simulink model "Navion_6DoF_10_auto_ascend_2023"  (R2024a)
settings: Solver=ode45  StartTime=0.0  StopTime=500  FixedStep=.01  MaxStep=.004  RelTol=1e-5  EnableMultiTasking=on
values from neighbouring files (symbols this model uses):
  ac = [0 0 0]    [Navion_Geom_temp.m]
  b = 33.4    [Navion_Geom_temp.m]
  cbar = 5.7    [Navion_Geom_temp.m]
  cda2 = 0.33    [Navion_Geom_temp.m]
  cdo = 0.05    [Navion_Geom_temp.m]
  cg = [0 0 0]    [Navion_Geom_temp.m]
  cla = 4.44    [Navion_Geom_temp.m]
  cladot = 0    [Navion_Geom_temp.m]
  clb = -0.074    [Navion_Geom_temp.m]
  clda = -0.134    [Navion_Geom_temp.m]
  clde = 0.355    [Navion_Geom_temp.m]
  cldr = 0.107    [Navion_Geom_temp.m]
  clo = 0.41    [Navion_Geom_temp.m]
  clp = -0.410    (= -0.41)    [Navion_Geom_temp.m]
  clq = 3.8    [Navion_Geom_temp.m]
  clr = 0.107    [Navion_Geom_temp.m]
  cma = -0.683    [Navion_Geom_temp.m]
  cmadot = -4.36    [Navion_Geom_temp.m]
  cmde = -0.923    [Navion_Geom_temp.m]
  cmq = -9.96    [Navion_Geom_temp.m]
  cnb = 0.071    [Navion_Geom_temp.m]
  cnda = -0.0035    [Navion_Geom_temp.m]
  cndr = -0.072    [Navion_Geom_temp.m]
  cnp = -0.0575    [Navion_Geom_temp.m]
  cnr = -0.125    [Navion_Geom_temp.m]
  cyb = -0.564    [Navion_Geom_temp.m]
  cydr = 0.157    [Navion_Geom_temp.m]
  eng = [0 0 0]    [Navion_Geom_temp.m]
  initalt = 5000    [Navion_Geom_temp.m]
  initbank = 0    [Navion_Geom_temp.m]
  initeast = 0    [Navion_Geom_temp.m]
  inithead = 0    [Navion_Geom_temp.m]
  initnorth = 0    [Navion_Geom_temp.m]
  initp = 0    [Navion_Geom_temp.m]
  initpitch = initw/initu    (= 0)    [Navion_Geom_temp.m]
  initq = 0    [Navion_Geom_temp.m]
  initr = 0    [Navion_Geom_temp.m]
  initu = 223    [Navion_Geom_temp.m]
  initv = 0    [Navion_Geom_temp.m]
  initw = 0    [Navion_Geom_temp.m]
  jx = 1048    [Navion_Geom_temp.m]
  jxz = 0    [Navion_Geom_temp.m]
  jy = 3000    [Navion_Geom_temp.m]
  jz = 3500    [Navion_Geom_temp.m]
  sw = 184    [Navion_Geom_temp.m]
  weight = 2750    [Navion_Geom_temp.m]
undefined symbols (not defined in the file or in its folder): Earth, WGS84
libraries: simulink_extras x9, slpidlib x6, aerolibfltsims x2, simulink x2, aerolibtransform2 x1, aerolibanimutils x1
(part 2 of 2)

== system Navion_6DoF_10_auto_ascend_2023/longitudinal autopilot/Descend ==
  note: this is desired rate of climb
  R/C : Inport
  Action Port : ActionPort  ActionPortLabel=elseif(u1 <100)
  Debugging : Constant  Value=2
  PID Controller : slpidlib/PID Controller  Controller=PID  Form=Parallel  TimeDomain=Continuous-time  UseExternalTs=off  SampleTime=-1  IntegratorMethod=Forward Euler  FilterMethod=Forward Euler  ControllerParametersSource=internal  P=1  I=1  UseKiTs=off  D=0  N=100  UseFilter=on  TunerSelectOption=Transfer Function Based (PID Tuner App)  InitialConditionSource=internal  InitialConditionForIntegrator=0  InitialConditionForFilter=0  DifferentiatorICPrevScaledInput=0  ExternalReset=none  TrackingMode=off  Kt=1  LimitOutput=off  SatLimitsSource=internal  UpperSaturationLimit=inf  LowerSaturationLimit=-inf  LinearizeAsGain=on  AntiWindupMode=none  Kb=1  LimitIntegrator=off  UpperIntegratorSaturationLimit=inf  LowerIntegratorSaturationLimit=-inf  POutMin=[]  POutMax=[]  IOutMin=[]  IOutMax=[]  DOutMin=[]  DOutMax=[]  NOutMin=[]  NOutMax=[]  SumOutMin=[]  SumOutMax=[]  SaturationOutMin=[]  SaturationOutMax=[]  PParamMin=[]  PParamMax=[]  IParamMin=[]  IParamMax=[]  DParamMin=[]  DParamMax=[]  NParamMin=[]  NParamMax=[]  KbParamMin=[]  KbParamMax=[]  KtParamMin=[]  KtParamMax=[]  KbOutMin=[]  KbOutMax=[]  KtOutMin=[]  KtOutMax=[]  IntegratorOutMin=[]  IntegratorOutMax=[]  FilterOutMin=[]  FilterOutMax=[]  SumI1OutMin=[]  SumI1OutMax=[]  SumI2OutMin=[]  SumI2OutMax=[]  SumI3OutMin=[]  SumI3OutMax=[]  SumI4OutMin=[]  SumI4OutMax=[]  SumDOutMin=[]  SumDOutMax=[]  DifferentiatorOutMin=[]  DifferentiatorOutMax=[]  FilterDiffOutCoefMin=[]  FilterDiffOutCoefMax=[]  ReciprocalOutMin=[]  ReciprocalOutMax=[]  SumDenOutMin=[]  SumDenOutMax=[]  SumNumOutMin=[]  SumNumOutMax=[]  DivideOutMin=[]  DivideOutMax=[]  UdiffTsProdOutMin=[]  UdiffTsProdOutMax=[]  NTsProdOutMin=[]  NTsProdOutMax=[]  UintegralTsProdOutMin=[]  UintegralTsProdOutMax=[]  UngainTsProdOutMin=[]  UngainTsProdOutMax=[]  ClampingZeroOutDataTypeStr=Inherit: Inherit via back propagation  ClampingZeroOutMin=[]  ClampingZeroOutMax=[]  FilterDenConstantOutDataTypeStr=Inherit: Inherit via back propagation  FilterDenConstantOutMin=[]  FilterDenConstantOutMax=[]  PCopyOutDataTypeStr=Inherit: Inherit via back propagation  PCopyOutMin=[]  PCopyOutMax=[]  NCopyOutDataTypeStr=Inherit: Inherit via back propagation  NCopyOutMin=[]  NCopyOutMax=[]  IntegratorContinuousStateAttributes=''  IntegratorStateMustResolveToSignalObject=off  IntegratorRTWStateStorageClass=Auto  FilterContinuousStateAttributes=''  FilterStateMustResolveToSignalObject=off  FilterRTWStateStorageClass=Auto  ParallelPVariant=InternalParameters  IdealPVariant=Disabled  IVariant=InternalParameters  DVariant=InternalParameters  IntegratorVariant=Continuous  SatVariant=Disabled  AWVariant=Passthrough  PCopyVariant=Disabled  TRVariant=Disabled  FdbkBlocksVariant=Forward  IdealPFdbkVariant=Disabled  SatFdbkVariant=Disabled  DerivativeFilterVariant=ContFilter  NVariant=InternalParameters  NCopyVariant=Disabled  FilterICVariant=InternalICsFilter  IntegratorICVariant=InternalICs  ExternalResetVariant=Disabled  TRSumVariant=Passthrough  SumFdbkVariant=Disabled  SumVariant=Sum_PID  TsampFilterVariant=InternalTs  TsampNgainVariant=Passthrough  TsampIntegralVariant=Disabled_SignalSpec  ExternalSaturationOutDataTypeStr=Inherit: Same as second input
  R/C_CMD : Constant  Value=-1
  Sum : Sum  Inputs=|+-
  del_e_auto : Outport
  Debug : Outport  Port=2
  wires:
  Debugging/1 -> Debug/1
  R/C_CMD/1 -> Sum/2
  PID Controller/1 -> del_e_auto/1
  Sum/1 -> PID Controller/1
  R/C/1 -> Sum/1

== system Navion_6DoF_10_auto_ascend_2023/longitudinal autopilot/Level ==
  h_err : Inport
  Action Port : ActionPort  ActionPortLabel=else
  Constant : Constant  Value=3
  PID Controller : slpidlib/PID Controller  Controller=PID  Form=Parallel  TimeDomain=Continuous-time  UseExternalTs=off  SampleTime=-1  IntegratorMethod=Forward Euler  FilterMethod=Forward Euler  ControllerParametersSource=internal  P=8.53679546434618e-05  I=3.54615014998628e-06  UseKiTs=off  D=0.000510671209456043  N=32.652227886903  UseFilter=on  TunerSelectOption=Transfer Function Based (PID Tuner App)  InitialConditionSource=internal  InitialConditionForIntegrator=0  InitialConditionForFilter=0  DifferentiatorICPrevScaledInput=0  ExternalReset=none  TrackingMode=off  Kt=1  LimitOutput=on  SatLimitsSource=internal  UpperSaturationLimit=.4363  LowerSaturationLimit=-.4363  LinearizeAsGain=off  AntiWindupMode=none  Kb=1  LimitIntegrator=off  UpperIntegratorSaturationLimit=inf  LowerIntegratorSaturationLimit=-inf  POutMin=[]  POutMax=[]  IOutMin=[]  IOutMax=[]  DOutMin=[]  DOutMax=[]  NOutMin=[]  NOutMax=[]  SumOutMin=[]  SumOutMax=[]  SaturationOutMin=[]  SaturationOutMax=[]  PParamMin=[]  PParamMax=[]  IParamMin=[]  IParamMax=[]  DParamMin=[]  DParamMax=[]  NParamMin=[]  NParamMax=[]  KbParamMin=[]  KbParamMax=[]  KtParamMin=[]  KtParamMax=[]  KbOutMin=[]  KbOutMax=[]  KtOutMin=[]  KtOutMax=[]  IntegratorOutMin=[]  IntegratorOutMax=[]  FilterOutMin=[]  FilterOutMax=[]  SumI1OutMin=[]  SumI1OutMax=[]  SumI2OutMin=[]  SumI2OutMax=[]  SumI3OutMin=[]  SumI3OutMax=[]  SumI4OutMin=[]  SumI4OutMax=[]  SumDOutMin=[]  SumDOutMax=[]  DifferentiatorOutMin=[]  DifferentiatorOutMax=[]  FilterDiffOutCoefMin=[]  FilterDiffOutCoefMax=[]  ReciprocalOutMin=[]  ReciprocalOutMax=[]  SumDenOutMin=[]  SumDenOutMax=[]  SumNumOutMin=[]  SumNumOutMax=[]  DivideOutMin=[]  DivideOutMax=[]  UdiffTsProdOutMin=[]  UdiffTsProdOutMax=[]  NTsProdOutMin=[]  NTsProdOutMax=[]  UintegralTsProdOutMin=[]  UintegralTsProdOutMax=[]  UngainTsProdOutMin=[]  UngainTsProdOutMax=[]  ClampingZeroOutDataTypeStr=Inherit: Inherit via back propagation  ClampingZeroOutMin=[]  ClampingZeroOutMax=[]  FilterDenConstantOutDataTypeStr=Inherit: Inherit via back propagation  FilterDenConstantOutMin=[]  FilterDenConstantOutMax=[]  PCopyOutDataTypeStr=Inherit: Inherit via back propagation  PCopyOutMin=[]  PCopyOutMax=[]  NCopyOutDataTypeStr=Inherit: Inherit via back propagation  NCopyOutMin=[]  NCopyOutMax=[]  IntegratorContinuousStateAttributes=''  IntegratorStateMustResolveToSignalObject=off  IntegratorRTWStateStorageClass=Auto  FilterContinuousStateAttributes=''  FilterStateMustResolveToSignalObject=off  FilterRTWStateStorageClass=Auto  ParallelPVariant=InternalParameters  IdealPVariant=Disabled  IVariant=InternalParameters  DVariant=InternalParameters  IntegratorVariant=Continuous  SatVariant=Enabled  AWVariant=Passthrough  PCopyVariant=Disabled  TRVariant=Disabled  FdbkBlocksVariant=Forward  IdealPFdbkVariant=Disabled  SatFdbkVariant=Disabled  DerivativeFilterVariant=ContFilter  NVariant=InternalParameters  NCopyVariant=Disabled  FilterICVariant=InternalICsFilter  IntegratorICVariant=InternalICs  ExternalResetVariant=Disabled  TRSumVariant=Passthrough  SumFdbkVariant=Disabled  SumVariant=Sum_PID  TsampFilterVariant=InternalTs  TsampNgainVariant=Passthrough  TsampIntegralVariant=Disabled_SignalSpec  ExternalSaturationOutDataTypeStr=Inherit: Same as second input
  del_e_auto : Outport
  Debug : Outport  Port=2
  wires:
  h_err/1 -> PID Controller/1
  PID Controller/1 -> del_e_auto/1  "Hal"
  Constant/1 -> Debug/1

== system Navion_6DoF_10_auto_ascend_2023/Aircraft_Dynamics/Aerodynamics/Aero Forces and Moments ==
  dyn(q) : Inport
  CD : Inport  Port=2
  CY : Inport  Port=3
  CL : Inport  Port=4
  Wind Para : Inport  Port=5
  Croll : Inport  Port=6
  CM : Inport  Port=7
  CN : Inport  Port=8
  Aerodynamic Forces : Subsystem
  Aerodynamic Moments : Subsystem
  Faero : Outport
  Maero : Outport  Port=2
  wires:
  dyn(q)/1 -> Aerodynamic Moments/1(dyn(q)), Aerodynamic Forces/5(dyn(q))
  CD/1 -> Aerodynamic Forces/1(CD)
  CY/1 -> Aerodynamic Forces/2(CY)
  CL/1 -> Aerodynamic Forces/3(CL)
  Wind Para/1 -> Aerodynamic Forces/4(Wind Para)
  Croll/1 -> Aerodynamic Moments/2(Croll)
  CM/1 -> Aerodynamic Moments/3(CM)
  CN/1 -> Aerodynamic Moments/4(CN)
  Aerodynamic Forces/1(FaeroBody) -> Faero/1
  Aerodynamic Moments/1(Maero) -> Maero/1

== system Navion_6DoF_10_auto_ascend_2023/Aircraft_Dynamics/Aerodynamics/CD ==
  Wind Parameters : Inport
  Controls : Inport  Port=2
  Mach No. : Inport  Port=3
  "   1" : Terminator
  "   6" : Terminator
  Get Alpha : Subsystem
  Math Function : Math  Operator=square  SignedPower=on
  Sum : Sum  SaturateOnIntegerOverflow=on
  cda2 : Gain  Gain=cda2  SaturateOnIntegerOverflow=on  OutDataTypeStr=Inherit: Same as input  ParamDataTypeStr=Inherit: Same as input
  cdo : Constant  Value=cdo
  CD : Outport
  wires:
  Wind Parameters/1 -> Get Alpha/1(windPar)
  Sum/1 -> CD/1
  Controls/1 -> "   6"/1
  Get Alpha/1(Alpha) -> Math Function/1
  Math Function/1 -> cda2/1
  cda2/1 -> Sum/2
  Mach No./1 -> "   1"/1
  cdo/1 -> Sum/1

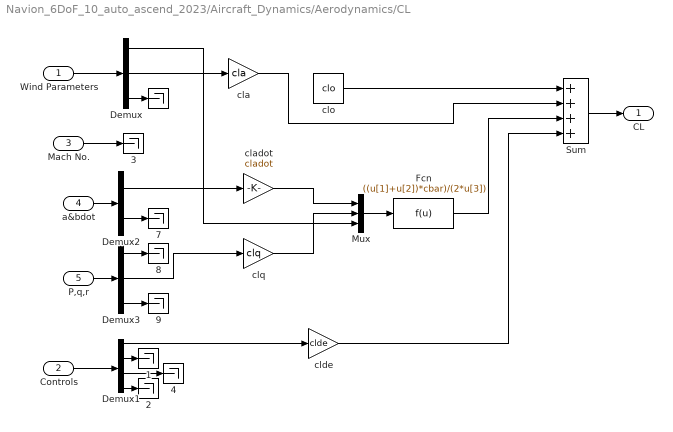
== system Navion_6DoF_10_auto_ascend_2023/Aircraft_Dynamics/Aerodynamics/CL ==
  Wind Parameters : Inport
  Controls : Inport  Port=2
  Mach No. : Inport  Port=3
  a&bdot : Inport  Port=4
  P,q,r : Inport  Port=5
     {,1..4,7..9} (8 alike) : Terminator
  Demux : Demux  Outputs=3
      settings: DisplayOption=none
  Demux1 : Demux
      settings: DisplayOption=none
  Demux2 : Demux  Outputs=2
      settings: DisplayOption=none
  Demux3 : Demux  Outputs=3
      settings: DisplayOption=none
  Fcn : Fcn  Expr=((u[1]+u[2])*cbar)/(2*u[3])
  Mux : Mux  Inputs=3
  Sum : Sum  Inputs=++++  SaturateOnIntegerOverflow=on
  cla : Gain  Gain=cla  SaturateOnIntegerOverflow=on  OutDataTypeStr=Inherit: Same as input  ParamDataTypeStr=Inherit: Same as input
  cladot : Gain  Gain=cladot  SaturateOnIntegerOverflow=on  OutDataTypeStr=Inherit: Same as input  ParamDataTypeStr=Inherit: Same as input
  clde : Gain  Gain=clde  SaturateOnIntegerOverflow=on  OutDataTypeStr=Inherit: Same as input  ParamDataTypeStr=Inherit: Same as input
  clo : Constant  Value=clo
  clq : Gain  Gain=clq  SaturateOnIntegerOverflow=on  OutDataTypeStr=Inherit: Same as input  ParamDataTypeStr=Inherit: Same as input
  CL : Outport
  wires:
  Mux/1 -> Fcn/1
  Demux/1 -> Mux/3
  clo/1 -> Sum/1
  Demux2/2 -> "   7"/1
  Demux3/1 -> "   8"/1
  Demux3/3 -> "   9"/1
  Wind Parameters/1 -> Demux/1
  Sum/1 -> CL/1
  Controls/1 -> Demux1/1
  a&bdot/1 -> Demux2/1
  P,q,r/1 -> Demux3/1
  Demux/3 -> "   "/1
  Demux1/4 -> "   2"/1
  cla/1 -> Sum/2
  Demux2/1 -> cladot/1
  cladot/1 -> Mux/1
  Demux/2 -> cla/1
  clq/1 -> Mux/2
  Mach No./1 -> "   3"/1
  Demux3/2 -> clq/1
  Demux1/1 -> clde/1
  Demux1/2 -> "   1"/1
  Demux1/3 -> "   4"/1
  Fcn/1 -> Sum/3
  clde/1 -> Sum/4

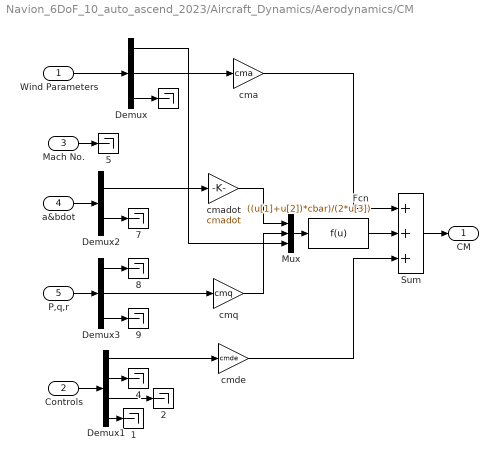
== system Navion_6DoF_10_auto_ascend_2023/Aircraft_Dynamics/Aerodynamics/CM ==
  Wind Parameters : Inport
  Controls : Inport  Port=2
  Mach No. : Inport  Port=3
  a&bdot : Inport  Port=4
  P,q,r : Inport  Port=5
     {,1..2,4..5,7..9} (8 alike) : Terminator
  Demux : Demux  Outputs=3
      settings: DisplayOption=none
  Demux1 : Demux
      settings: DisplayOption=none
  Demux2 : Demux  Outputs=2
      settings: DisplayOption=none
  Demux3 : Demux  Outputs=3
      settings: DisplayOption=none
  Fcn : Fcn  Expr=((u[1]+u[2])*cbar)/(2*u[3])
  Mux : Mux  Inputs=3
  Sum : Sum  Inputs=+++  SaturateOnIntegerOverflow=on
  cma : Gain  Gain=cma  SaturateOnIntegerOverflow=on  OutDataTypeStr=Inherit: Same as input  ParamDataTypeStr=Inherit: Same as input
  cmadot : Gain  Gain=cmadot  SaturateOnIntegerOverflow=on  OutDataTypeStr=Inherit: Same as input  ParamDataTypeStr=Inherit: Same as input
  cmde : Gain  Gain=cmde  SaturateOnIntegerOverflow=on  OutDataTypeStr=Inherit: Same as input  ParamDataTypeStr=Inherit: Same as input
  cmq : Gain  Gain=cmq  SaturateOnIntegerOverflow=on  OutDataTypeStr=Inherit: Same as input  ParamDataTypeStr=Inherit: Same as input
  CM : Outport
  wires:
  Demux2/2 -> "   7"/1
  Demux3/1 -> "   8"/1
  Demux3/3 -> "   9"/1
  Wind Parameters/1 -> Demux/1
  Sum/1 -> CM/1
  Controls/1 -> Demux1/1
  a&bdot/1 -> Demux2/1
  P,q,r/1 -> Demux3/1
  Demux/3 -> "   "/1
  Demux1/4 -> "   1"/1
  Demux1/3 -> "   2"/1
  Demux/2 -> cma/1
  cmadot/1 -> Mux/1
  cmq/1 -> Mux/2
  Mux/1 -> Fcn/1
  Demux1/2 -> "   4"/1
  Mach No./1 -> "   5"/1
  Demux/1 -> Mux/3
  cma/1 -> Sum/1
  Demux1/1 -> cmde/1
  Demux2/1 -> cmadot/1
  Demux3/2 -> cmq/1
  Fcn/1 -> Sum/2
  cmde/1 -> Sum/3

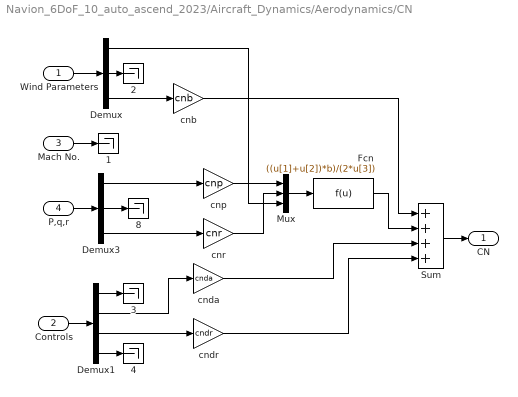
== system Navion_6DoF_10_auto_ascend_2023/Aircraft_Dynamics/Aerodynamics/CN ==
  Wind Parameters : Inport
  Controls : Inport  Port=2
  Mach No. : Inport  Port=3
  P,q,r : Inport  Port=4
     {1..4,8} (5 alike) : Terminator
  Demux : Demux  Outputs=3
      settings: DisplayOption=none
  Demux1 : Demux
      settings: DisplayOption=none
  Demux3 : Demux  Outputs=3
      settings: DisplayOption=none
  Fcn : Fcn  Expr=((u[1]+u[2])*b)/(2*u[3])
  Mux : Mux  Inputs=3
  Sum : Sum  Inputs=++++  SaturateOnIntegerOverflow=on
  cnb : Gain  Gain=cnb  SaturateOnIntegerOverflow=on  OutDataTypeStr=Inherit: Same as input  ParamDataTypeStr=Inherit: Same as input
  cnda : Gain  Gain=cnda  SaturateOnIntegerOverflow=on  OutDataTypeStr=Inherit: Same as input  ParamDataTypeStr=Inherit: Same as input
  cndr : Gain  Gain=cndr  SaturateOnIntegerOverflow=on  OutDataTypeStr=Inherit: Same as input  ParamDataTypeStr=Inherit: Same as input
  cnp : Gain  Gain=cnp  SaturateOnIntegerOverflow=on  OutDataTypeStr=Inherit: Same as input  ParamDataTypeStr=Inherit: Same as input
  cnr : Gain  Gain=cnr  SaturateOnIntegerOverflow=on  OutDataTypeStr=Inherit: Same as input  ParamDataTypeStr=Inherit: Same as input
  CN : Outport
  wires:
  Mux/1 -> Fcn/1
  Demux/2 -> "   2"/1
  Wind Parameters/1 -> Demux/1
  Sum/1 -> CN/1
  Controls/1 -> Demux1/1
  P,q,r/1 -> Demux3/1
  Demux3/2 -> "   8"/1
  cnb/1 -> Sum/1
  Mach No./1 -> "   1"/1
  Demux/3 -> cnb/1
  Demux/1 -> Mux/3
  Demux3/1 -> cnp/1
  cnp/1 -> Mux/1
  Demux3/3 -> cnr/1
  cnr/1 -> Mux/2
  Demux1/2 -> cnda/1
  Demux1/3 -> cndr/1
  Fcn/1 -> Sum/2
  cnda/1 -> Sum/3
  cndr/1 -> Sum/4
  Demux1/1 -> "   3"/1
  Demux1/4 -> "   4"/1

== system Navion_6DoF_10_auto_ascend_2023/Aircraft_Dynamics/Aerodynamics/CY ==
  Wind Parameters : Inport
  Controls : Inport  Port=2
  Mach No. : Inport  Port=3
  P,q,r : Inport  Port=4
     {2,7..12} (7 alike) : Terminator
  Demux : Demux  Outputs=3
      settings: DisplayOption=none
  Demux1 : Demux
      settings: DisplayOption=none
  Sum : Sum  SaturateOnIntegerOverflow=on
  cyb : Gain  Gain=cyb  SaturateOnIntegerOverflow=on  OutDataTypeStr=Inherit: Same as input  ParamDataTypeStr=Inherit: Same as input
  cydr : Gain  Gain=cydr  SaturateOnIntegerOverflow=on  OutDataTypeStr=Inherit: Same as input  ParamDataTypeStr=Inherit: Same as input
  CY : Outport
  wires:
  Demux/2 -> "   9"/1
  Wind Parameters/1 -> Demux/1
  Sum/1 -> CY/1
  Controls/1 -> Demux1/1
  P,q,r/1 -> "   8"/1
  Demux/3 -> cyb/1
  Mach No./1 -> "   2"/1
  Demux1/3 -> cydr/1
  Demux1/1 -> "   10"/1
  Demux1/2 -> "   7"/1
  Demux1/4 -> "   11"/1
  cyb/1 -> Sum/1
  cydr/1 -> Sum/2
  Demux/1 -> "   12"/1

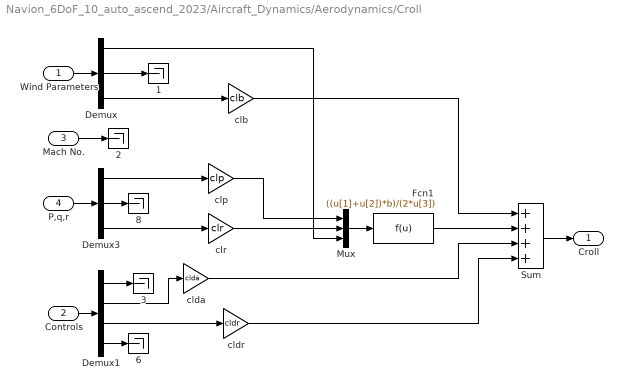
== system Navion_6DoF_10_auto_ascend_2023/Aircraft_Dynamics/Aerodynamics/Croll ==
  Wind Parameters : Inport
  Controls : Inport  Port=2
  Mach No. : Inport  Port=3
  P,q,r : Inport  Port=4
     {1..3,6,8} (5 alike) : Terminator
  Demux : Demux  Outputs=3
      settings: DisplayOption=none
  Demux1 : Demux
      settings: DisplayOption=none
  Demux3 : Demux  Outputs=3
      settings: DisplayOption=none
  Fcn1 : Fcn  Expr=((u[1]+u[2])*b)/(2*u[3])
  Mux : Mux  Inputs=3
  Sum : Sum  Inputs=++++  SaturateOnIntegerOverflow=on
  clb : Gain  Gain=clb  SaturateOnIntegerOverflow=on  OutDataTypeStr=Inherit: Same as input  ParamDataTypeStr=Inherit: Same as input
  clda : Gain  Gain=clda  SaturateOnIntegerOverflow=on  OutDataTypeStr=Inherit: Same as input  ParamDataTypeStr=Inherit: Same as input
  cldr : Gain  Gain=cldr  SaturateOnIntegerOverflow=on  OutDataTypeStr=Inherit: Same as input  ParamDataTypeStr=Inherit: Same as input
  clp : Gain  Gain=clp  SaturateOnIntegerOverflow=on  OutDataTypeStr=Inherit: Same as input  ParamDataTypeStr=Inherit: Same as input
  clr : Gain  Gain=clr  SaturateOnIntegerOverflow=on  OutDataTypeStr=Inherit: Same as input  ParamDataTypeStr=Inherit: Same as input
  Croll : Outport
  wires:
  Mux/1 -> Fcn1/1
  Demux/2 -> "   1"/1
  Wind Parameters/1 -> Demux/1
  Sum/1 -> Croll/1
  Controls/1 -> Demux1/1
  P,q,r/1 -> Demux3/1
  Demux3/2 -> "   8"/1
  Demux1/1 -> "   3"/1
  clp/1 -> Mux/1
  clb/1 -> Sum/1
  Demux/1 -> Mux/3
  Demux/3 -> clb/1
  Mach No./1 -> "   2"/1
  Demux3/1 -> clp/1
  Fcn1/1 -> Sum/2
  Demux3/3 -> clr/1
  clr/1 -> Mux/2
  Demux1/4 -> "   6"/1
  Demux1/2 -> clda/1
  Demux1/3 -> cldr/1
  clda/1 -> Sum/3
  cldr/1 -> Sum/4

== system Navion_6DoF_10_auto_ascend_2023/Aircraft_Dynamics/Equations of motion numerical integration /Flat Earth Navigation ==
  note: 1  roll
      | 2  pitch
      | 3  yaw
      | 4 u
      | 5 v
      | 6 w
  Euler Angles : Inport
  Velocity : Inport  Port=2
  Alt : Integrator  InitialCondition=initalt
  Alttitude Dot : Fcn  Expr=u[4] * sin(u[2]) - u[5] * sin(u[1]) * cos(u[2]) - u[6] * cos(u[1]) * cos(u[2])
  Demux : Demux  Outputs=3
      settings: DisplayOption=none
  Demux1 : Demux  Outputs=3
      settings: DisplayOption=none
  East : Integrator  InitialCondition=initeast
  East Dot : Fcn  Expr=u[4] * cos(u[2])* sin(u[3]) + u[5] * (cos(u[1])*cos(u[3]) + sin(u[1])*sin(u[2])*sin(u[3])) + u[6] * (-sin(u[1])*cos(u[3])+cos(u[1])*sin(u[2])*sin(u[3]))
  Mux : Mux  Inputs=6
  Mux1 : Mux  Inputs=3
  North : Integrator  InitialCondition=initnorth
  North Dot : Fcn  Expr=u[4] * cos(u[2]) * cos(u[3]) + u[5]*(-cos(u[1])*sin(u[3])+sin(u[1])*sin(u[2])*sin(u[3]))+u[6]*(sin(u[1])*sin(u[3])+cos(u[1])*sin(u[2])*cos(u[3]))
  Position : Outport
  R/C : Outport  Port=2
  wires:
  Euler Angles/1 -> Demux/1
  Velocity/1 -> Demux1/1
  Demux/1 -> Mux/1
  Demux/2 -> Mux/2
  Demux/3 -> Mux/3
  Demux1/1 -> Mux/4
  Demux1/2 -> Mux/5
  Demux1/3 -> Mux/6
  Mux/1 -> East Dot/1, Alttitude Dot/1, North Dot/1
  East Dot/1 -> East/1
  North Dot/1 -> North/1
  Alttitude Dot/1 -> R/C/1, Alt/1
  East/1 -> Mux1/2
  North/1 -> Mux1/1
  Alt/1 -> Mux1/3
  Mux1/1 -> Position/1

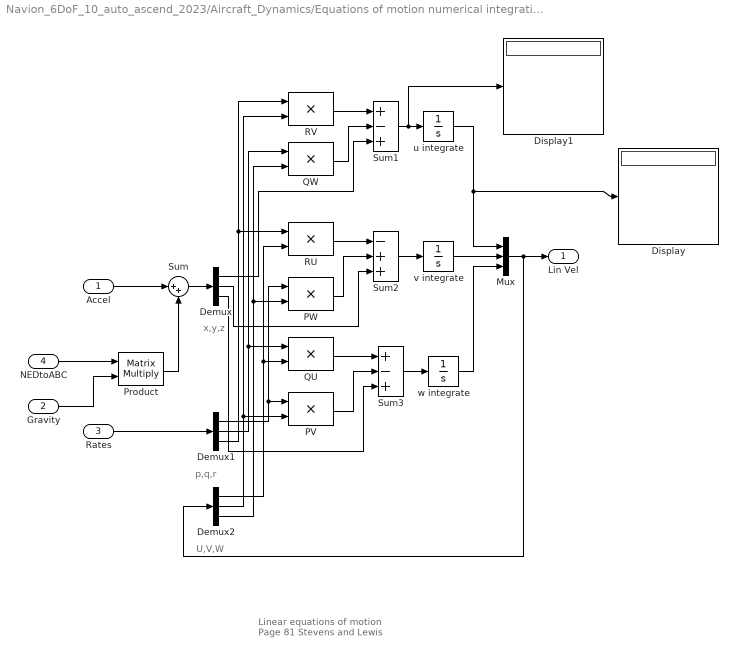
== system Navion_6DoF_10_auto_ascend_2023/Aircraft_Dynamics/Equations of motion numerical integration /Force Equations ==
  note: U,V,W
  note: p,q,r
  note: x,y,z
  note: Linear equations of motion
      | Page 81 Stevens and Lewis
  Accel : Inport
  Gravity : Inport  Port=2
  Rates : Inport  Port=3
  NEDtoABC : Inport  Port=4
  Demux : Demux  Outputs=3
      settings: DisplayOption=none
  Demux1 : Demux  Outputs=3
      settings: DisplayOption=none
  Demux2 : Demux  Outputs=3
      settings: DisplayOption=none
  Display : Display
  Display1 : Display
  Mux : Mux  Inputs=3
  PV : Product  SaturateOnIntegerOverflow=on  OutDataTypeStr=Inherit: Same as first input
  PW : Product  SaturateOnIntegerOverflow=on  OutDataTypeStr=Inherit: Same as first input
  Product : Product  Multiplication=Matrix(*)  SaturateOnIntegerOverflow=on  OutDataTypeStr=Inherit: Same as first input
  QU : Product  SaturateOnIntegerOverflow=on  OutDataTypeStr=Inherit: Same as first input
  QW : Product  SaturateOnIntegerOverflow=on  OutDataTypeStr=Inherit: Same as first input
  RU : Product  SaturateOnIntegerOverflow=on  OutDataTypeStr=Inherit: Same as first input
  RV : Product  SaturateOnIntegerOverflow=on  OutDataTypeStr=Inherit: Same as first input
  Sum : Sum  Inputs=|++  SaturateOnIntegerOverflow=on
  Sum1 : Sum  Inputs=+-+  SaturateOnIntegerOverflow=on
  Sum2 : Sum  Inputs=-++  SaturateOnIntegerOverflow=on
  Sum3 : Sum  Inputs=+-+  SaturateOnIntegerOverflow=on
  u integrate : Integrator  InitialCondition=initu
  v integrate : Integrator  InitialCondition=initv
  w integrate : Integrator  InitialCondition=initw
  Lin Vel : Outport
  wires:
  Sum/1 -> Demux/1
  Accel/1 -> Sum/1
  Rates/1 -> Demux1/1
  Mux/1 -> Demux2/1, Lin Vel/1
  Demux1/3 -> RV/1, RU/1
  Demux2/2 -> RV/2, PV/2
  RV/1 -> Sum1/1
  Demux1/2 -> QW/1, QU/1
  Demux2/3 -> QW/2, PW/2
  QW/1 -> Sum1/2
  Demux/1 -> Sum1/3
  Demux2/1 -> RU/2, QU/2
  RU/1 -> Sum2/1
  Demux1/1 -> PV/1, PW/1
  PW/1 -> Sum2/2
  Demux/2 -> Sum2/3
  QU/1 -> Sum3/1
  PV/1 -> Sum3/2
  Demux/3 -> Sum3/3
  Gravity/1 -> Product/2
  NEDtoABC/1 -> Product/1
  Product/1 -> Sum/2
  Sum1/1 -> u integrate/1, Display1/1
  Sum2/1 -> v integrate/1
  Sum3/1 -> w integrate/1
  u integrate/1 -> Mux/1, Display/1
  v integrate/1 -> Mux/2
  w integrate/1 -> Mux/3

== system Navion_6DoF_10_auto_ascend_2023/Aircraft_Dynamics/Equations of motion numerical integration /Gravity Model ==
  Constant : Constant  Value=0
  Constant1 : Constant  Value=32.2
  Mux : Mux  Inputs=3
  Gravity : Outport
  wires:
  Constant/1 -> Mux/1, Mux/2
  Constant1/1 -> Mux/3
  Mux/1 -> Gravity/1

== system Navion_6DoF_10_auto_ascend_2023/Aircraft_Dynamics/Equations of motion numerical integration /Inert-body ==
  Euler : Inport
  11 : Fcn  Expr=cos(u[2])*cos(u[3])
  12 : Fcn  Expr=-cos(u[1])*sin(u[3])+sin(u[1])*sin(u[2])*cos(u[3])
  13 : Fcn  Expr=sin(u[1])*sin(u[3])+cos(u[1])*sin(u[2])*cos(u[3])
  21 : Fcn  Expr=cos(u[2])*sin(u[3])
  22 : Fcn  Expr=cos(u[1])*cos(u[3]) + sin(u[1])*sin(u[2])*sin(u[3])
  23 : Fcn  Expr=-sin(u[1])*cos(u[3])+cos(u[1])*sin(u[2])*sin(u[3])
  31 : Fcn  Expr=-sin(u[2])
  32 : Fcn  Expr=sin(u[1]) * cos(u[2])
  33 : Fcn  Expr=cos(u[1])*cos(u[2])
  Matrix Concatenation : Concatenate  NumInputs=3  Mode=Multidimensional array
  Matrix Concatenation1 : Concatenate  NumInputs=3  Mode=Multidimensional array
  Matrix Concatenation2 : Concatenate  NumInputs=3  Mode=Multidimensional array
  Matrix Concatenation3 : Concatenate  NumInputs=3  Mode=Multidimensional array  ConcatenateDimension=2
  NEDtoBC : Outport
  wires:
  Euler/1 -> 11/1, 12/1, 13/1, 21/1, 22/1, 23/1, 31/1, 33/1, 32/1
  12/1 -> Matrix Concatenation/2
  11/1 -> Matrix Concatenation/1
  13/1 -> Matrix Concatenation/3
  22/1 -> Matrix Concatenation1/2
  21/1 -> Matrix Concatenation1/1
  23/1 -> Matrix Concatenation1/3
  32/1 -> Matrix Concatenation2/2
  31/1 -> Matrix Concatenation2/1
  33/1 -> Matrix Concatenation2/3
  Matrix Concatenation1/1 -> Matrix Concatenation3/2
  Matrix Concatenation/1 -> Matrix Concatenation3/1
  Matrix Concatenation2/1 -> Matrix Concatenation3/3
  Matrix Concatenation3/1 -> NEDtoBC/1

== system Navion_6DoF_10_auto_ascend_2023/Aircraft_Dynamics/Equations of motion numerical integration /Kinematic Equiations ==
  note: 1  p
      | 2  q
      | 3  r
      | 4  bank
      | 5 pitch
      | 6 Yaw
  Rates : Inport
  2pi Bound : Subsystem  mask(2pi bound){}
      mask help: Bounds the input angle to [0, 2pi]. When 0 bound is exceeded the output wraps back to 2pi; when the 2pi bound is exceeded the output wraps back to 0.
      mask Help:
      | Bounds the input angle to [0, 2pi]. When 0 bound is exceeded the output wraps back to 2pi; when the 2pi bound is exceeded the output wraps back to 0.
      | <P><B>Input:</B> any angle in radians, from -Inf to Inf;</P>
      | <P><B>Output:</B> an angle in radians between zero and 2pi.</P>
  Demux : Demux  Outputs=3
      settings: DisplayOption=none
  Demux1 : Demux  Outputs=3
      settings: DisplayOption=none
  Demux2 : Demux  Outputs=3
      settings: DisplayOption=none
  Mux : Mux  Inputs=6
  Mux1 : Mux  Inputs=3
  Mux2 : Mux  Inputs=3
  Yaw rate : Fcn  Expr=(u[2] * sin(u[4]) + u[3] * cos(u[4]))/cos(u[5])
  bank : Integrator  InitialCondition=initbank
  heading : Integrator  InitialCondition=inithead
  pi Bound : Subsystem  mask(pi bound){}
      mask help: Bounds the input angle to [-pi, pi]. When -pi bound is exceeded the output wraps back to pi; when the pi bound is exceeded the output wraps back to -pi.
      mask Help:
      | Bounds the input angle to [-pi, pi]. When -pi bound is exceeded the output wraps back to pi; when the pi bound is exceeded the output wraps back to -pi.
      | <P><B>Input:</B> any angle in radians, from -Inf to Inf;</P>
      | <P><B>Output:</B> an angle in radians between -pi and pi.</P>
  pi Bound1 : Subsystem  mask(pi bound){}
      mask help: Bounds the input angle to [-pi, pi]. When -pi bound is exceeded the output wraps back to pi; when the pi bound is exceeded the output wraps back to -pi.
      mask Help:
      | Bounds the input angle to [-pi, pi]. When -pi bound is exceeded the output wraps back to pi; when the pi bound is exceeded the output wraps back to -pi.
      | <P><B>Input:</B> any angle in radians, from -Inf to Inf;</P>
      | <P><B>Output:</B> an angle in radians between -pi and pi.</P>
  pitch : Integrator  InitialCondition=initpitch
  pitch rate : Fcn  Expr=u[2] *cos(u[4]) - u[3] * sin(u[4])
  roll rate : Fcn  Expr=u[1] + tan(u[5])*(u[2]*sin(u[4])+u[3]*cos(u[4]))
  Euler angles : Outport
  wires:
  Rates/1 -> Demux/1
  Demux/2 -> Mux/2
  Demux/3 -> Mux/3
  Demux1/1 -> Mux/4
  Demux1/2 -> Mux/5
  Demux1/3 -> Mux/6
  Demux/1 -> Mux/1
  Mux/1 -> roll rate/1, Yaw rate/1, pitch rate/1
  Demux2/3 -> 2pi Bound/1(In)
  Demux2/2 -> pi Bound/1(In)
  Demux2/1 -> pi Bound1/1(In)
  Mux2/1 -> Euler angles/1
  pi Bound/1(Out) -> Mux2/2
  pi Bound1/1(Out) -> Mux2/1
  2pi Bound/1(Out) -> Mux2/3
  pitch rate/1 -> pitch/1
  roll rate/1 -> bank/1
  Yaw rate/1 -> heading/1
  bank/1 -> Mux1/1
  pitch/1 -> Mux1/2
  heading/1 -> Mux1/3
  Mux1/1 -> Demux2/1, Demux1/1

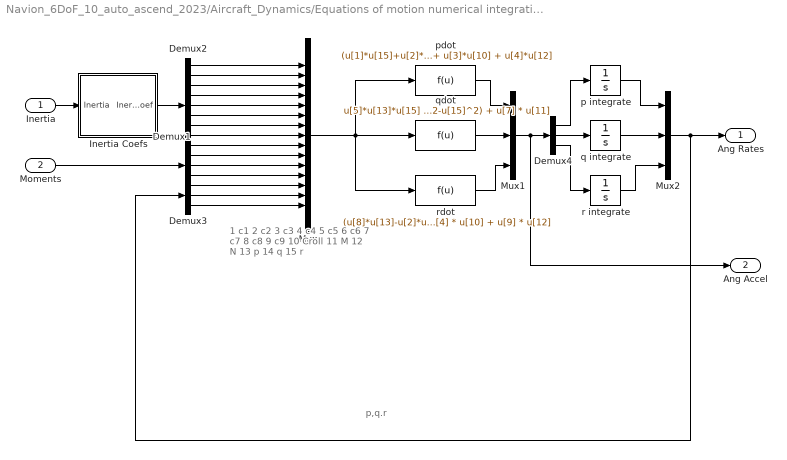
== system Navion_6DoF_10_auto_ascend_2023/Aircraft_Dynamics/Equations of motion numerical integration /Moment Equations ==
  note: 1   c1
      | 2   c2
      | 3   c3
      | 4  c4
      | 5  c5
      | 6  c6
      | 7  c7
      | 8  c8
      | 9  c9
      | 10 Croll
      | 11  M
      | 12  N
      | 13  p
      | 14  q
      | 15  r
  note: p,q.r
  Inertia : Inport
  Moments : Inport  Port=2
  Demux1 : Demux  Outputs=3
      settings: DisplayOption=none
  Demux2 : Demux  Outputs=9
      settings: DisplayOption=none
  Demux3 : Demux  Outputs=3
      settings: DisplayOption=none
  Demux4 : Demux  Outputs=3
      settings: DisplayOption=none
  Inertia Coefs : Subsystem
  Mux : Mux  Inputs=15
  Mux1 : Mux  Inputs=3
  Mux2 : Mux  Inputs=3
  p integrate : Integrator  InitialCondition=initp
  pdot : Fcn  Expr=(u[1]*u[15]+u[2]*u[13])*u[14] + u[3]*u[10] + u[4]*u[12]
  q integrate : Integrator  InitialCondition=initq
  qdot : Fcn  Expr=u[5]*u[13]*u[15] - u[6]*(u[13]^2-u[15]^2) + u[7] * u[11]
  r integrate : Integrator  InitialCondition=initr
  rdot : Fcn  Expr=(u[8]*u[13]-u[2]*u[15]) * u[14] + u[4] * u[10] + u[9] * u[12]
  Ang Rates : Outport
  Ang Accel : Outport  Port=2
  wires:
  Inertia/1 -> Inertia Coefs/1(Inertia)
  Moments/1 -> Demux1/1
  Inertia Coefs/1(Iner Coef) -> Demux2/1
  Demux2/1 -> Mux/1
  Demux2/2 -> Mux/2
  Demux2/3 -> Mux/3
  Demux2/4 -> Mux/4
  Demux2/5 -> Mux/5
  Demux2/6 -> Mux/6
  Demux2/7 -> Mux/7
  Demux2/8 -> Mux/8
  Demux2/9 -> Mux/9
  Demux1/1 -> Mux/10
  Demux1/2 -> Mux/11
  Demux1/3 -> Mux/12
  Demux3/1 -> Mux/13
  Demux3/2 -> Mux/14
  Demux3/3 -> Mux/15
  Mux/1 -> pdot/1, qdot/1, rdot/1
  qdot/1 -> Mux1/2
  pdot/1 -> Mux1/1
  rdot/1 -> Mux1/3
  Mux1/1 -> Ang Accel/1, Demux4/1
  Demux4/1 -> p integrate/1
  Demux4/2 -> q integrate/1
  Demux4/3 -> r integrate/1
  Mux2/1 -> Ang Rates/1, Demux3/1
  p integrate/1 -> Mux2/1
  q integrate/1 -> Mux2/2
  r integrate/1 -> Mux2/3

== system Navion_6DoF_10_auto_ascend_2023/Aircraft_Dynamics/Linear Acc and Moments/Cross Prod Moment due Leng ==
  Vec 1 : Inport
  Vec 2 : Inport  Port=2
  Check prob not zero : Constant  Value=0
  Demux : Demux  Outputs=3
      settings: DisplayOption=none
  J axis : Fcn  Expr=u[4]*u[3] - u[6]*u[1]
  Mux : Mux  Inputs=6
  Mux1 : Mux  Inputs=3
  i axis : Fcn  Expr=u[6]*u[2] - u[5]*u[3]
  k axis : Fcn  Expr=u[5]*u[1] - u[4]*u[2]
  X Prod : Outport
  wires:
  Vec 2/1 -> Mux/4
  Vec 1/1 -> Demux/1
  Demux/1 -> Mux/1
  Check prob not zero/1 -> Mux/5, Mux/6
  Demux/3 -> Mux/3
  Demux/2 -> Mux/2
  Mux/1 -> i axis/1, J axis/1, k axis/1
  J axis/1 -> Mux1/2
  i axis/1 -> Mux1/1
  k axis/1 -> Mux1/3
  Mux1/1 -> X Prod/1

== system Navion_6DoF_10_auto_ascend_2023/Aircraft_Dynamics/Linear Acc and Moments/Cross Prod Moment due to Aero ==
  Vec 1 : Inport
  Vec 2 : Inport  Port=2
  Demux : Demux  Outputs=3
      settings: DisplayOption=none
  Demux1 : Demux  Outputs=3
      settings: DisplayOption=none
  J axis : Fcn  Expr=u[4]*u[3] - u[6]*u[1]
  Mux : Mux  Inputs=6
  Mux1 : Mux  Inputs=3
  i axis : Fcn  Expr=u[6]*u[2] - u[5]*u[3]
  k axis : Fcn  Expr=u[5]*u[1] - u[4]*u[2]
  X Prod : Outport
  wires:
  Vec 2/1 -> Demux1/1
  Vec 1/1 -> Demux/1
  Demux/1 -> Mux/1
  Demux1/3 -> Mux/6
  Demux1/2 -> Mux/5
  Demux1/1 -> Mux/4
  Demux/3 -> Mux/3
  Demux/2 -> Mux/2
  Mux/1 -> i axis/1, J axis/1, k axis/1
  J axis/1 -> Mux1/2
  i axis/1 -> Mux1/1
  k axis/1 -> Mux1/3
  Mux1/1 -> X Prod/1

== system Navion_6DoF_10_auto_ascend_2023/Aircraft_Dynamics/Aerodynamics/Aero Forces and Moments/Aerodynamic Forces ==
  CD : Inport
  CY : Inport  Port=2
  CL : Inport  Port=3
  Wind Para : Inport  Port=4
  dyn(q) : Inport  Port=5
  Body to Wind : Subsystem
  Demux : Demux  Outputs=3
      settings: DisplayOption=none
  Gain : Gain  Gain=-1  SaturateOnIntegerOverflow=on  OutDataTypeStr=Inherit: Same as input  ParamDataTypeStr=Inherit: Same as input
  Gain1 : Gain  Gain=-1  SaturateOnIntegerOverflow=on  OutDataTypeStr=Inherit: Same as input  ParamDataTypeStr=Inherit: Same as input
  Gain2 : Gain  Gain=sw  SaturateOnIntegerOverflow=on  OutDataTypeStr=Inherit: Same as input  ParamDataTypeStr=Inherit: Same as input
  Math Function : Math  Operator=transpose  SignedPower=on
  Mux : Mux  Inputs=3
  Product : Product  SaturateOnIntegerOverflow=on  OutDataTypeStr=Inherit: Same as first input
  Product1 : Product  Multiplication=Matrix(*)  SaturateOnIntegerOverflow=on  OutDataTypeStr=Inherit: Same as first input
  Terminator : Terminator
  FaeroBody : Outport
  wires:
  Gain/1 -> Mux/1
  Gain1/1 -> Mux/3
  Mux/1 -> Product/1
  Gain2/1 -> Product/2
  CD/1 -> Gain/1
  CY/1 -> Mux/2
  CL/1 -> Gain1/1
  dyn(q)/1 -> Gain2/1
  Wind Para/1 -> Demux/1
  Demux/1 -> Terminator/1
  Body to Wind/1(Smatrix) -> Math Function/1
  Math Function/1 -> Product1/1
  Product/1 -> Product1/2
  Product1/1 -> FaeroBody/1
  Demux/2 -> Body to Wind/1(Alpha)
  Demux/3 -> Body to Wind/2(Beta)

== system Navion_6DoF_10_auto_ascend_2023/Aircraft_Dynamics/Aerodynamics/Aero Forces and Moments/Aerodynamic Moments ==
  dyn(q) : Inport
  Croll : Inport  Port=2
  CM : Inport  Port=3
  CN : Inport  Port=4
  Mux : Mux  Inputs=2
  Mux1 : Mux  Inputs=2
  Mux2 : Mux  Inputs=2
  Mux3 : Mux  Inputs=3
  Pitch : Fcn  Expr=u[1] * sw * cbar * u[2]
  Roll : Fcn  Expr=u[1] * sw * b * u[2]
  Yaw : Fcn  Expr=u[1] * sw * b * u[2]
  Maero : Outport
  wires:
  Mux/1 -> Roll/1
  Mux1/1 -> Pitch/1
  Mux2/1 -> Yaw/1
  Pitch/1 -> Mux3/2
  Roll/1 -> Mux3/1
  Yaw/1 -> Mux3/3
  dyn(q)/1 -> Mux/1, Mux1/1, Mux2/1
  Croll/1 -> Mux/2
  CM/1 -> Mux1/2
  CN/1 -> Mux2/2
  Mux3/1 -> Maero/1

== system Navion_6DoF_10_auto_ascend_2023/Aircraft_Dynamics/Aerodynamics/CD/Get Alpha ==
  windPar : Inport
  "   " : Terminator
  "   1" : Terminator
  Demux : Demux  Outputs=3
      settings: DisplayOption=none
  Alpha : Outport
  wires:
  Demux/1 -> "   1"/1
  Demux/3 -> "   "/1
  windPar/1 -> Demux/1
  Demux/2 -> Alpha/1

== system Navion_6DoF_10_auto_ascend_2023/Aircraft_Dynamics/Equations of motion numerical integration /Kinematic Equiations/2pi Bound ==
  In : Inport
  2pi : Constant  Value=2*pi
  Math Function : Math  Operator=mod  SignedPower=on
  Out : Outport
  wires:
  Math Function/1 -> Out/1
  2pi/1 -> Math Function/2
  In/1 -> Math Function/1

== system Navion_6DoF_10_auto_ascend_2023/Aircraft_Dynamics/Equations of motion numerical integration /Kinematic Equiations/pi Bound ==
  In : Inport
  2pi : Constant  Value=2*pi
  Math Function : Math  Operator=mod  SignedPower=on
  Sum1 : Sum  Inputs=|+-  InputSameDT=on  SaturateOnIntegerOverflow=on  OutDataTypeStr=Inherit: Same as first input
  Sum2 : Sum  Inputs=|++  InputSameDT=on  SaturateOnIntegerOverflow=on  OutDataTypeStr=Inherit: Same as first input
  pi : Constant  Value=pi
  Out : Outport
  wires:
  Sum1/1 -> Out/1
  pi/1 -> Sum1/2, Sum2/2
  Sum2/1 -> Math Function/1
  In/1 -> Sum2/1
  2pi/1 -> Math Function/2
  Math Function/1 -> Sum1/1

== system Navion_6DoF_10_auto_ascend_2023/Aircraft_Dynamics/Equations of motion numerical integration /Kinematic Equiations/pi Bound1 ==
  In : Inport
  2pi : Constant  Value=2*pi
  Math Function : Math  Operator=mod  SignedPower=on
  Sum1 : Sum  Inputs=|+-  InputSameDT=on  SaturateOnIntegerOverflow=on  OutDataTypeStr=Inherit: Same as first input
  Sum2 : Sum  Inputs=|++  InputSameDT=on  SaturateOnIntegerOverflow=on  OutDataTypeStr=Inherit: Same as first input
  pi : Constant  Value=pi
  Out : Outport
  wires:
  Sum1/1 -> Out/1
  pi/1 -> Sum1/2, Sum2/2
  Sum2/1 -> Math Function/1
  In/1 -> Sum2/1
  2pi/1 -> Math Function/2
  Math Function/1 -> Sum1/1

== system Navion_6DoF_10_auto_ascend_2023/Aircraft_Dynamics/Equations of motion numerical integration /Moment Equations/Inertia Coefs ==
  note: Jx,Jy,Jz,Jxz
  note: Inertia Coefficeents
      | Page 80 Stevens and Lewis
  Inertia : Inport
  Mux : Mux  Inputs=9
  c1 : Fcn  Expr=((u[2]-u[3])*u[3] - u[4]^2)/(u[1]*u[3]-u[4]^2)
  c2 : Fcn  Expr=((u[1]-u[2]+u[3])*u[4])/(u[1]*u[3]-u[4]^2)
  c3 : Fcn  Expr=u[3]/(u[1]*u[3]-u[4]^2)
  c4 : Fcn  Expr=u[4]/(u[1]*u[3]-u[4]^2)
  c5 : Fcn  Expr=(u[3]-u[1])/u[2]
  c6 : Fcn  Expr=u[4]/u[2]
  c7 : Fcn  Expr=1/u[2]
  c8 : Fcn  Expr=(u[1]*(u[1]-u[2])+u[4]^2)/(u[1]*u[3]-u[4]^2)
  c9 : Fcn  Expr=u[1]/(u[1]*u[3]-u[4]^2)
  Iner Coef : Outport
  wires:
  Inertia/1 -> c1/1, c2/1, c3/1, c4/1, c5/1, c6/1, c7/1, c9/1, c8/1
  c1/1 -> Mux/1
  c2/1 -> Mux/2
  c3/1 -> Mux/3
  c4/1 -> Mux/4
  c5/1 -> Mux/5
  c6/1 -> Mux/6
  c7/1 -> Mux/7
  c8/1 -> Mux/8
  c9/1 -> Mux/9
  Mux/1 -> Iner Coef/1

== system Navion_6DoF_10_auto_ascend_2023/Aircraft_Dynamics/Aerodynamics/Aero Forces and Moments/Aerodynamic Forces/Body to Wind ==
  note: This transforms any arbitrary vector from body axis to wind axis.
      | Page 63  Stevens and Lewis
  Alpha : Inport
  Beta : Inport  Port=2
  -ca sb : Fcn  Expr=-1 * cos(u[1]) * sin(u[2])
  -sa : Fcn  Expr=-1 * sin(u[1])
  -sa sb : Fcn  Expr="-1 * sin(u[1])  * sin(u[2])"
  Fcn8 : Fcn  Expr=cos(u[1])
  Matrix Concatenation : Concatenate  NumInputs=3  Mode=Multidimensional array
  Matrix Concatenation1 : Concatenate  NumInputs=3  Mode=Multidimensional array
  Matrix Concatenation2 : Concatenate  NumInputs=3  Mode=Multidimensional array  ConcatenateDimension=2
  Matrix Concatenation3 : Concatenate  NumInputs=3  Mode=Multidimensional array
  Mux1 : Mux  Inputs=2
  ca cb : Fcn  Expr="cos(u[1]) *  cos(u[2])"
  cb : Fcn  Expr=cos(u[2])
  sa cb : Fcn  Expr=sin(u[1]) * cos(u[2])
  sb : Fcn  Expr=sin(u[2])
  zero : Fcn  Expr=u[1] * 0
  Smatrix : Outport
  wires:
  Matrix Concatenation/1 -> Matrix Concatenation2/1
  Matrix Concatenation1/1 -> Matrix Concatenation2/2
  Matrix Concatenation3/1 -> Matrix Concatenation2/3
  -ca sb/1 -> Matrix Concatenation/2
  ca cb/1 -> Matrix Concatenation/1
  -sa/1 -> Matrix Concatenation/3
  zero/1 -> Matrix Concatenation1/3
  sb/1 -> Matrix Concatenation1/1
  cb/1 -> Matrix Concatenation1/2
  sa cb/1 -> Matrix Concatenation3/1
  -sa sb/1 -> Matrix Concatenation3/2
  Fcn8/1 -> Matrix Concatenation3/3
  Mux1/1 -> ca cb/1, -ca sb/1, -sa/1, sb/1, cb/1, zero/1, sa cb/1, -sa sb/1, Fcn8/1
  Alpha/1 -> Mux1/1
  Beta/1 -> Mux1/2
  Matrix Concatenation2/1 -> Smatrix/1

== matlab function Navion_6DoF_10_auto_ascend_2023/Waypoint calculator ==
  data: position input; relative_heading output; distance output; waypoint input
function [relative_heading,distance] = heading_desired_fcn(position,waypoint)
%[north,east,down]
x_distance = waypoint(1)-position(1);
y_distance = waypoint(2)-position(2);
direction_vector = [x_distance,y_distance];
distance = norm(direction_vector);
%fprintf("true heading is %.3f deg",rad2deg(atan2(y_distance,x_distance)));
relative_heading = rad2deg(atan2(y_distance,x_distance));
%desired_heading = deg2rad(angle_deg);

== matlab function Navion_6DoF_10_auto_ascend_2023/Desired & current heading to error/MATLAB Function ==
  data: heading input; error output; desired input
function error = fcn(heading,desired)


heading_vec = [sin(heading),cos(heading)];
desired_vec = [sin(desired),cos(desired)];
% Compute the dot product between the vectors
dot_product = dot(heading_vec, desired_vec);
% Compute the cross product (in 2D, it returns a scalar)
cross_product = heading_vec(1) * desired_vec(2) - heading_vec(2) * desired_vec(1);

% Compute the angle between the vectors (in radians)
error = acos(dot_product);
if cross_product < 0
    error= -error;  % Desired is to the left of heading
end

== matlab function Navion_6DoF_10_auto_ascend_2023/MATLAB Function ==
  data: old_signal input; XYZ input; signal output; waypoint input; distance output
function [signal,distance]  = fcn(old_signal,XYZ,waypoint)

distance = norm(waypoint - XYZ);
signal=old_signal;
if distance < 100
    fprintf("WAYPOINT REACHED")
    signal = old_signal + 1
end

== matlab function Navion_6DoF_10_auto_ascend_2023/Xbox Controller/MATLAB Function1 ==
  data: u input; y output
function y = fcn(u)
%#codegen

y = u-.5;

== matlab function Navion_6DoF_10_auto_ascend_2023/Xbox Controller/MATLAB Function2 ==
  data: u input; y output
function y = fcn(u)
%#codegen

if u == 16
y=1;

elseif u == 32
y=-1;
elseif u == 48
y=0;
else
y=0;
end
end

== matlab function Navion_6DoF_10_auto_ascend_2023/Xbox Controller/MATLAB Function3 ==
  data: u input; y output
function y = fcn(u)
%#codegen

y = u-.5;

== matlab function Navion_6DoF_10_auto_ascend_2023/Xbox Controller/MATLAB Function4 ==
  data: int input; y output; trigger input
function y = throttle_control(int,trigger)
%#codegen

if int >= 1 && trigger >=0
y= 0;

elseif int <= 0 && trigger <=0
y= 0;

else
y=1;
end
end

== matlab function Navion_6DoF_10_auto_ascend_2023/Xbox Controller/MATLAB Function5 ==
  data: u input; y output
function y = roll_to_ailron(u)
%this assumes that your max ailron is 25 deg
if sqrt(u^2) >= 0.08 %this is just the deadzone of my stick, and helps xbox stick drift

    y=-1*sign(u)*25*u^2;
else
    y=0;
end

end

== matlab function Navion_6DoF_10_auto_ascend_2023/Xbox Controller/MATLAB Function6 ==
  data: u input; y output
function y = pitch_to_elevator(u)
%this assumes that your max ailron is 25 deg
if sqrt(u^2) >= 0.08 %this is just the deadzone of my stick, and helps xbox stick drift

    y=sign(u)*25*u^2;
else
    y=0;
end

end
